simulink model "Sim_Trayect"  (R2024b)
settings: Solver=VariableStepAuto  StartTime=0.0  StopTime=2  RelTol=1e-3
settings Model: Creator=javier  LastModifiedBy=javier

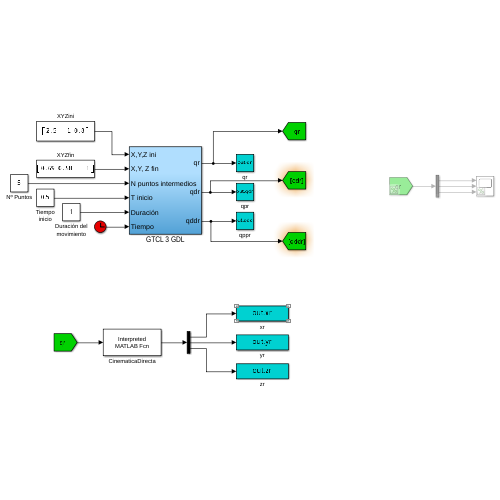
[thumbnail: Simulink's stored preview of the top-level diagram]
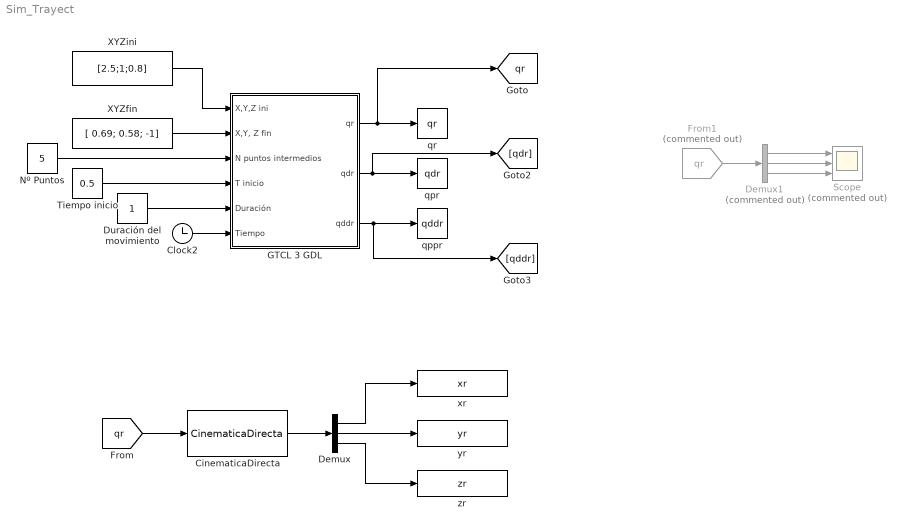
== system Sim_Trayect ==
  CinematicaDirecta : MATLABFcn  MATLABFcn=CinematicaDirecta  OutputDimensions=3
  Clock2 : Clock
  Demux : Demux  Outputs=3
  Demux1 : Demux  Commented=on  Outputs=3
  Duración del movimiento : Constant
  From1 : From  Commented=on  GotoTag=qr  TagVisibility=global
  GTCL 3 GDL : Subsystem
  Nº Puntos : Constant  Value=5
  Scope : Scope  Commented=on  NumInputPorts=3
  Tiempo inicio : Constant  Value=0.5
  XYZfin : Constant  Value=[ 0.69; 0.58; -1]
  XYZini : Constant  Value=[2.5;1;0.8]
  qppr : ToWorkspace  VariableName=qddr  SampleTime=-1
  qpr : ToWorkspace  VariableName=qdr  SampleTime=-1
  qr : ToWorkspace  VariableName=qr  SampleTime=-1
  xr : ToWorkspace  VariableName=xr  SampleTime=-1
  yr : ToWorkspace  VariableName=yr  SampleTime=-1
  zr : ToWorkspace  VariableName=zr  SampleTime=-1
  tag scope: qr=global
  wires:
  Duración del movimiento/1 -> GTCL 3 GDL/5(Duración)
  XYZfin/1 -> GTCL 3 GDL/2("X,Y, Z fin")
  Nº Puntos/1 -> GTCL 3 GDL/3(N puntos intermedios)
  Tiempo inicio/1 -> GTCL 3 GDL/4(T inicio)
  GTCL 3 GDL/1(qr) -> [qr], qr/1
  GTCL 3 GDL/3(qddr) -> [qddr], qppr/1
  Clock2/1 -> GTCL 3 GDL/6(Tiempo)
  GTCL 3 GDL/2(qdr) -> [qdr], qpr/1
  XYZini/1 -> GTCL 3 GDL/1(X,Y,Z ini)
  [qr] -> CinematicaDirecta/1
  CinematicaDirecta/1 -> Demux/1
  Demux/1 -> xr/1
  Demux/3 -> zr/1
  Demux/2 -> yr/1
  From1/1 -> Demux1/1
  Demux1/1 -> Scope/1
  Demux1/2 -> Scope/2
  Demux1/3 -> Scope/3

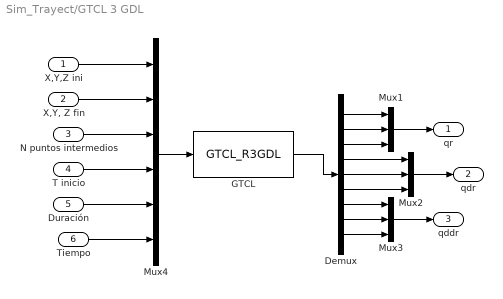
== system Sim_Trayect/GTCL 3 GDL ==
  X,Y,Z ini : Inport
  "X,Y, Z fin" : Inport  Port=2
  N puntos intermedios : Inport  Port=3
  T inicio : Inport  Port=4
  Duración : Inport  Port=5
  Tiempo : Inport  Port=6
  Demux : Demux  Outputs=9
  GTCL : MATLABFcn  MATLABFcn=GTCL_R3GDL  OutputDimensions=9
  Mux1 : Mux  Inputs=3
  Mux2 : Mux  Inputs=3
  Mux3 : Mux  Inputs=3
  Mux4 : Mux  Inputs=6
  qr : Outport
  qdr : Outport  Port=2
  qddr : Outport  Port=3
  wires:
  Mux1/1 -> qr/1
  Mux4/1 -> GTCL/1
  X,Y,Z ini/1 -> Mux4/1
  "X,Y, Z fin"/1 -> Mux4/2
  N puntos intermedios/1 -> Mux4/3
  T inicio/1 -> Mux4/4
  Duración/1 -> Mux4/5
  Tiempo/1 -> Mux4/6
  GTCL/1 -> Demux/1
  Demux/1 -> Mux1/1
  Demux/2 -> Mux1/2
  Demux/3 -> Mux1/3
  Mux2/1 -> qdr/1
  Demux/4 -> Mux2/1
  Demux/5 -> Mux2/2
  Demux/6 -> Mux2/3
  Mux3/1 -> qddr/1
  Demux/7 -> Mux3/1
  Demux/8 -> Mux3/2
  Demux/9 -> Mux3/3
